simulink model "Expt3_19EE30018"  (R2020b)
settings: Solver=VariableStepAuto  StartTime=0.0  StopTime=0.1  MaxStep=1e-6  RelTol=1e-3
libraries: powerlib x13, eeGeneralControl x1, simulink x1
settings Model: Creator=HP  LastModifiedBy=HP

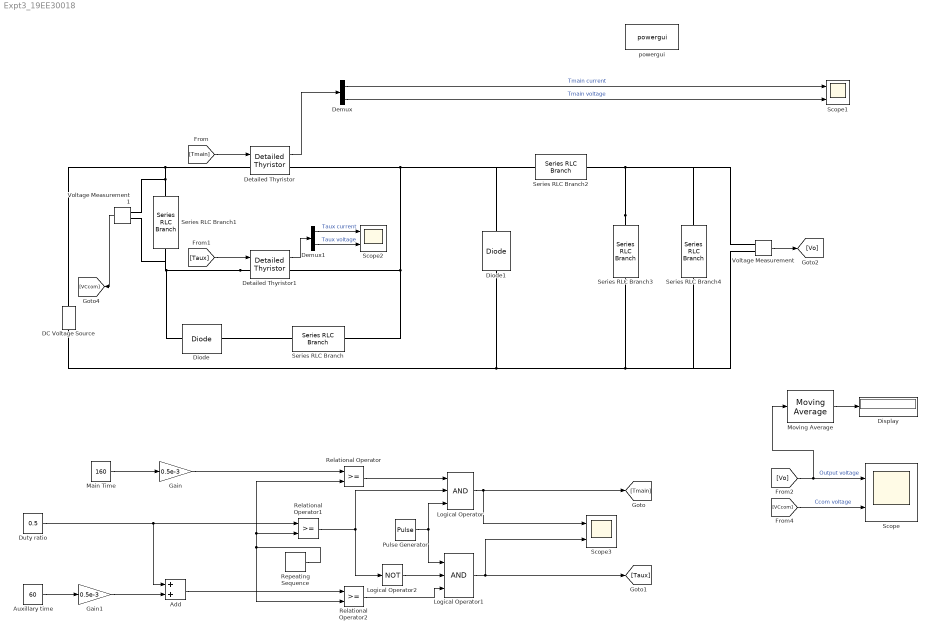
== system Expt3_19EE30018 ==
  Add : Sum
  Auxillary time : Constant  Value=60
  DC Voltage Source : powerlib/Electrical Sources/DC Voltage Source  Amplitude=1000  Measurements=None
  Demux : Demux  Outputs=2
      settings: DisplayOption=none
  Demux1 : Demux  Outputs=2
      settings: DisplayOption=none
  Detailed Thyristor : powerlib/Power Electronics/Detailed Thyristor  Ron=1e-6  Lon=1e-3  Vf=0  IL=0.1  Tq=100e-6  IC=0  Rs=inf  Cs=0  Measurements=on
      settings: SourceProductBaseCode=PS
  Detailed Thyristor1 : powerlib/Power Electronics/Detailed Thyristor  Ron=1e-6  Lon=1e-3  Vf=0  IL=0.1  Tq=100e-6  IC=0  Rs=inf  Cs=0  Measurements=on
      settings: SourceProductBaseCode=PS
  Diode : powerlib/Power Electronics/Diode  Ron=1e-6  Lon=0  Vf=0  IC=0  UseSnubber=0  Rs=inf  Cs=0  Measurements=off
  Diode1 : powerlib/Power Electronics/Diode  Ron=1e-6  Lon=0  Vf=0  IC=0  UseSnubber=0  Rs=inf  Cs=0  Measurements=off
  Display : Display
  Duty ratio : Constant  Value=0.5
  Gain : Gain  Gain=0.5e-3
  Gain1 : Gain  Gain=0.5e-3
  Logical Operator : Logic  Inputs=3  AllPortsSameDT=off  OutDataTypeStr=boolean
  Logical Operator1 : Logic  Inputs=3  AllPortsSameDT=off  OutDataTypeStr=boolean
  Logical Operator2 : Logic  Operator=NOT  AllPortsSameDT=off  OutDataTypeStr=boolean
  Main Time : Constant  Value=160
  Moving Average : eeGeneralControl/Moving Average  VariantControl=Variant1  LabelModeActiveChoice=Continuous  f=500  x0=0  Ts=0
      settings: SourceProductBaseCode=PS
  Pulse Generator : DiscretePulseGenerator  PulseType=Time based  Period=20e-6  PulseWidth=50
  Relational Operator : RelationalOperator  OutDataTypeStr=boolean  RndMeth=Simplest
  Relational Operator1 : RelationalOperator  OutDataTypeStr=boolean  RndMeth=Simplest
  Relational Operator2 : RelationalOperator  OutDataTypeStr=boolean  RndMeth=Simplest
  Repeating Sequence : simulink/Sources/Repeating Sequence  rep_seq_t=[0 1]/500  rep_seq_y=[0 1]
  Scope{,1..3} (4 alike) : Scope  NumInputPorts=2
  Series RLC Branch : powerlib/Elements/Series RLC Branch  LConnTagsString=__new0  RConnTagsString=__new0  BranchType=L  Resistance=1  Inductance=260e-6  SetiL0=off  InitialCurrent=0  Capacitance=1e-6  Setx0=off  InitialVoltage=0  Measurements=None
  Series RLC Branch1 : powerlib/Elements/Series RLC Branch  LConnTagsString=__new0  RConnTagsString=__new0  BranchType=C  Resistance=1  Inductance=1e-3  SetiL0=off  InitialCurrent=0  Capacitance=3e-6  Setx0=on  InitialVoltage=1000  Measurements=None
  Series RLC Branch2 : powerlib/Elements/Series RLC Branch  LConnTagsString=__new0  RConnTagsString=__new0  BranchType=L  Resistance=1  Inductance=24e-3  SetiL0=off  InitialCurrent=0  Capacitance=1e-6  Setx0=off  InitialVoltage=0  Measurements=None
  Series RLC Branch3 : powerlib/Elements/Series RLC Branch  LConnTagsString=__new0  RConnTagsString=__new0  BranchType=C  Resistance=1  Inductance=1e-3  SetiL0=off  InitialCurrent=0  Capacitance=330e-6  Setx0=off  InitialVoltage=0  Measurements=None
  Series RLC Branch4 : powerlib/Elements/Series RLC Branch  LConnTagsString=__new0  RConnTagsString=__new0  BranchType=R  Resistance=30  Inductance=1e-3  SetiL0=off  InitialCurrent=0  Capacitance=1e-6  Setx0=off  InitialVoltage=0  Measurements=None
  Voltage Measurement : powerlib/Measurements/Voltage Measurement  PhasorSimulation=off  OutputType=Complex  PSBequivalent=0
  Voltage Measurement1 : powerlib/Measurements/Voltage Measurement  PhasorSimulation=off  OutputType=Complex  PSBequivalent=0
  powergui : powerlib/powergui  Priority=1  SimulationMode=Continuous  SampleTime=50e-6  frequency=60  Iterations=50  frequencyindice=0  Pbase=100e6  ErrMax=1e-4  UnitsV=kV  UnitsW=MW  buscounter=0  FunctionMessages=off  echomessages=off  EnableUseOfTLC=off  CurrentSourceSwitches=off  DisableSnubberDevices=off  DisableRonSwitches=off  DisableVfSwitches=off  DisplayEquations=off  AutomaticDiscreteSolvers=off  SolverType=Tustin/Backward Euler (TBE)  Interpol=off  ExternalGateDelay=off  methode=off  Ts=100  x0status=blocks  SPID=on  SwTol=0  HookPort=off  NonlinearTolerance=1e-4  nMaxIteration=100  ContinueOnMaxIteration=off  RestoreLinks=warning  ResistiveCurrentMeasurement=off  Frange=[0:2:500]  Ylog=off  Xlog=on  ShowGrid=off  save=off  variable=ZData  structure=0  ZoomFFT=off  StartTime=0.0  cycles=1  DisplayStyle=1  fundamental=60  FreqAxis=off  MaxFrequency=1000  frequencyindicesteady=1  RmsSteady=1  display=off
  wires:
  Detailed Thyristor1/1 -> Demux1/1
  [Tmain] -> Detailed Thyristor/1
  Detailed Thyristor/1 -> Demux/1
  Voltage Measurement1/1 -> [VCcom]
  Demux1/1 -> Scope2/1  "Taux current"
  Demux/1 -> Scope1/1  "Tmain current"
  Demux/2 -> Scope1/2  "Tmain voltage"
  Voltage Measurement/1 -> [Vo]
  [Taux] -> Detailed Thyristor1/1
  Demux1/2 -> Scope2/2  "Taux voltage"
  [Vo] -> Moving Average/1, Scope/1  "Output voltage"
  Logical Operator2/1 -> Logical Operator1/2
  Gain/1 -> Relational Operator/1
  Logical Operator1/1 -> Scope3/2, [Taux]
  Duty ratio/1 -> Add/1, Relational Operator1/1
  Logical Operator/1 -> Scope3/1, [Tmain]
  [VCcom] -> Scope/2  "Ccom voltage"
  Auxillary time/1 -> Gain1/1
  Relational Operator1/1 -> Logical Operator/2, Logical Operator2/1
  Pulse Generator/1 -> Logical Operator1/1, Logical Operator/3
  Repeating Sequence/1 -> Relational Operator2/2, Relational Operator/2, Relational Operator1/2
  Main Time/1 -> Gain/1
  Gain1/1 -> Add/2
  Add/1 -> Relational Operator2/1
  Relational Operator/1 -> Logical Operator/1
  Relational Operator2/1 -> Logical Operator1/3
  Moving Average/1 -> Display/1
  connections:
  Series RLC Branch3/RConn1 -- Diode1/LConn1 -- DC Voltage Source/LConn1 -- Series RLC Branch4/RConn1 -- Voltage Measurement/LConn2
  Detailed Thyristor1/LConn1 -- Diode/RConn1 -- Voltage Measurement1/LConn2 -- Series RLC Branch1/RConn1
  Detailed Thyristor/RConn1 -- Detailed Thyristor1/RConn1 -- Series RLC Branch/LConn1 -- Series RLC Branch2/LConn1 -- Diode1/RConn1
  Series RLC Branch1/LConn1 -- DC Voltage Source/RConn1 -- Detailed Thyristor/LConn1 -- Voltage Measurement1/LConn1
  Series RLC Branch3/LConn1 -- Series RLC Branch2/RConn1 -- Series RLC Branch4/LConn1 -- Voltage Measurement/LConn1
  Diode/LConn1 -- Series RLC Branch/RConn1
